simulink model "Utkarsh_2005574_W2_P4"  (R2020b)
settings: Solver=ode45  StartTime=0.0  StopTime=0.08  RelTol=1e-3
PostLoadFcn:
  | J=3.2284e-6;
  | b=3.5077e-6;
  | K=0.0274;
  | R=4;
  | L=2.75e-6;
  | 
  | Kp=40.6275;
  | Ki=331.2128;
  | Kd=0.4934;
InitFcn:
  | J=3.2284e-6;
  | b=3.5077e-6;
  | K=0.0274;
  | R=4;
  | L=2.75e-6;
  | 
  | Kp=40.6275;
  | Ki=331.2128;
  | Kd=0.4934;
settings Model: Creator=home  LastModifiedBy=home

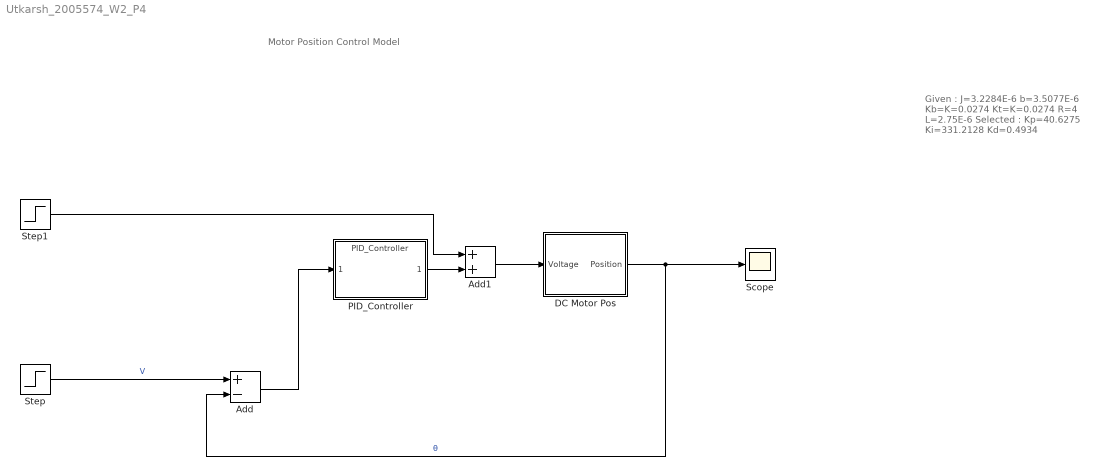
== system Utkarsh_2005574_W2_P4 ==
  note: Motor Position Control Model
  note: Given :
      | J=3.2284E-6
      | b=3.5077E-6
      | Kb=K=0.0274
      | Kt=K=0.0274
      | R=4
      | L=2.75E-6
      |
      | Selected :
      | Kp=40.6275
      | Ki=331.2128
      | Kd=0.4934
  Add : Sum  Inputs=+-
  Add1 : Sum
  DC Motor Pos : Subsystem
  PID_Controller : ModelReference  ModelNameDialog=PID_Controller  SimulationMode=Normal  ModelReferenceVersion=1.11
  Scope : Scope
  Step : Step  Time=0  SampleTime=0
  Step1 : Step  Time=0.03  SampleTime=0
  wires:
  Step/1 -> Add/1  "V"
  DC Motor Pos/1(Position) -> Add/2, Scope/1  "θ"
  Add/1 -> PID_Controller/1
  PID_Controller/1 -> Add1/2
  Add1/1 -> DC Motor Pos/1(Voltage)
  Step1/1 -> Add1/1

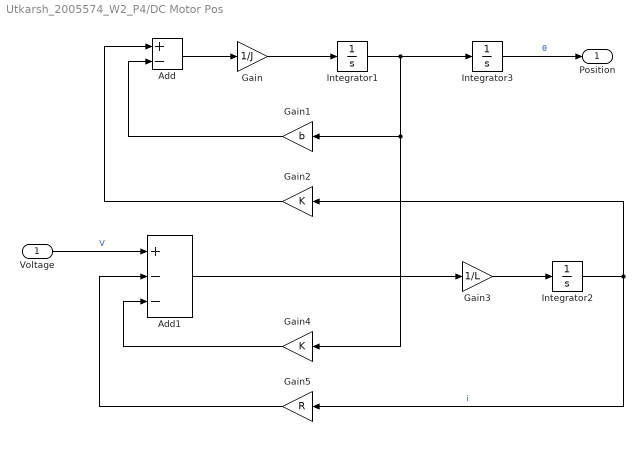
== system Utkarsh_2005574_W2_P4/DC Motor Pos ==
  Voltage : Inport
  Add : Sum  Inputs=+-
  Add1 : Sum  Inputs=+--
  Gain : Gain  Gain=1/J
  Gain1 : Gain  Gain=b
  Gain2 : Gain  Gain=K
  Gain3 : Gain  Gain=1/L
  Gain4 : Gain  Gain=K
  Gain5 : Gain  Gain=R
  Integrator1 : Integrator
  Integrator2 : Integrator
  Integrator3 : Integrator
  Position : Outport  VectorParamsAs1DForOutWhenUnconnected=off
  wires:
  Gain3/1 -> Integrator2/1
  Integrator1/1 -> Integrator3/1, Gain4/1, Gain1/1
  Integrator2/1 -> Gain5/1, Gain2/1  "i"
  Add/1 -> Gain/1
  Gain1/1 -> Add/2
  Gain/1 -> Integrator1/1
  Gain5/1 -> Add1/2
  Gain2/1 -> Add/1
  Gain4/1 -> Add1/3
  Add1/1 -> Gain3/1
  Voltage/1 -> Add1/1  "V"
  Integrator3/1 -> Position/1  "θ"
